simulink model "mainmodel"  (R2023b)
settings: Solver=FixedStepAuto  StartTime=0.0  StopTime=inf  RelTol=1e-3  EnableMultiTasking=on
libraries: vexarmcortexlib x26, simulink_extras x4, vexcommonlib x3
(part 2 of 2)

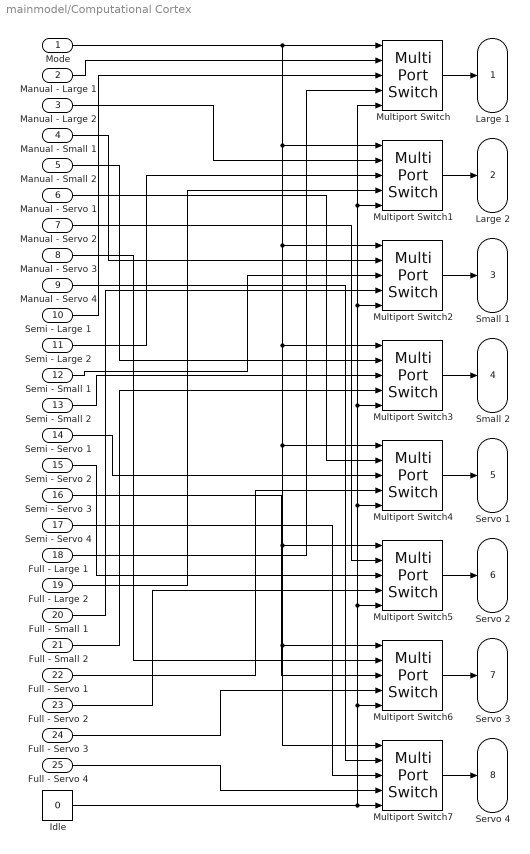
== system mainmodel/Computational Cortex ==
  Mode : Inport
  Manual - Large 1 : Inport  Port=2
  Manual - Large 2 : Inport  Port=3
  Manual - Small 1 : Inport  Port=4
  Manual - Small 2 : Inport  Port=5
  Manual - Servo 1 : Inport  Port=6
  Manual - Servo 2 : Inport  Port=7
  Manual - Servo 3 : Inport  Port=8
  Manual - Servo 4 : Inport  Port=9
  Semi - Large 1 : Inport  Port=10
  Semi - Large 2 : Inport  Port=11
  Semi - Small 1 : Inport  Port=12
  Semi - Small 2 : Inport  Port=13
  Semi - Servo 1 : Inport  Port=14
  Semi - Servo 2 : Inport  Port=15
  Semi - Servo 3 : Inport  Port=16
  Semi - Servo 4 : Inport  Port=17
  Full - Large 1 : Inport  Port=18
  Full - Large 2 : Inport  Port=19
  Full - Small 1 : Inport  Port=20
  Full - Small 2 : Inport  Port=21
  Full - Servo 1 : Inport  Port=22
  Full - Servo 2 : Inport  Port=23
  Full - Servo 3 : Inport  Port=24
  Full - Servo 4 : Inport  Port=25
  Idle : Constant  Value=0
  Multiport Switch{,1..7} (8 alike) : MultiPortSwitch  Inputs=4  SaturateOnIntegerOverflow=off  InputSameDT=off
  Large 1 : Outport
  Large 2 : Outport  Port=2
  Small 1 : Outport  Port=3
  Small 2 : Outport  Port=4
  Servo 1 : Outport  Port=5
  Servo 2 : Outport  Port=6
  Servo 3 : Outport  Port=7
  Servo 4 : Outport  Port=8
  wires:
  Multiport Switch/1 -> Large 1/1
  Multiport Switch1/1 -> Large 2/1
  Multiport Switch3/1 -> Small 2/1
  Multiport Switch2/1 -> Small 1/1
  Multiport Switch5/1 -> Servo 2/1
  Multiport Switch4/1 -> Servo 1/1
  Multiport Switch7/1 -> Servo 4/1
  Multiport Switch6/1 -> Servo 3/1
  Idle/1 -> Multiport Switch/5, Multiport Switch1/5, Multiport Switch2/5, Multiport Switch3/5, Multiport Switch4/5, Multiport Switch5/5, Multiport Switch6/5, Multiport Switch7/5
  Full - Servo 4/1 -> Multiport Switch7/4
  Full - Servo 3/1 -> Multiport Switch6/4
  Full - Servo 2/1 -> Multiport Switch5/4
  Full - Servo 1/1 -> Multiport Switch4/4
  Full - Small 2/1 -> Multiport Switch3/4
  Full - Small 1/1 -> Multiport Switch2/4
  Full - Large 2/1 -> Multiport Switch1/4
  Full - Large 1/1 -> Multiport Switch/4
  Semi - Servo 4/1 -> Multiport Switch7/3
  Semi - Servo 3/1 -> Multiport Switch6/3
  Semi - Servo 2/1 -> Multiport Switch5/3
  Semi - Servo 1/1 -> Multiport Switch4/3
  Semi - Small 2/1 -> Multiport Switch3/3
  Semi - Small 1/1 -> Multiport Switch2/3
  Semi - Large 2/1 -> Multiport Switch1/3
  Semi - Large 1/1 -> Multiport Switch/3
  Manual - Servo 4/1 -> Multiport Switch7/2
  Manual - Servo 3/1 -> Multiport Switch6/2
  Manual - Servo 2/1 -> Multiport Switch5/2
  Manual - Servo 1/1 -> Multiport Switch4/2
  Manual - Small 2/1 -> Multiport Switch3/2
  Manual - Small 1/1 -> Multiport Switch2/2
  Manual - Large 2/1 -> Multiport Switch1/2
  Manual - Large 1/1 -> Multiport Switch/2
  Mode/1 -> Multiport Switch3/1, Multiport Switch4/1, Multiport Switch7/1, Multiport Switch6/1, Multiport Switch5/1, Multiport Switch2/1, Multiport Switch1/1, Multiport Switch/1

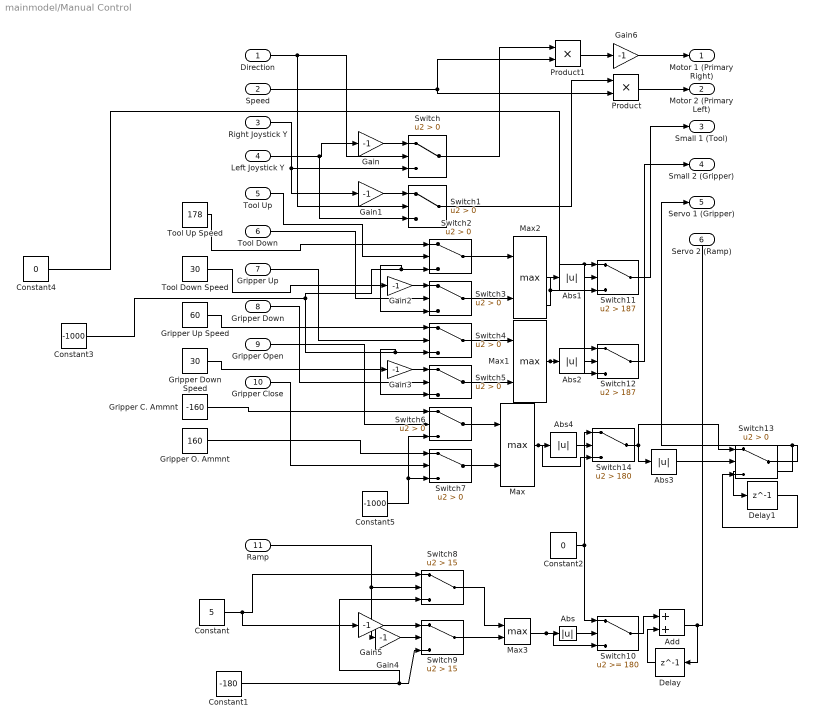
== system mainmodel/Manual Control ==
  Direction : Inport
  Speed : Inport  Port=2
  Right Joystick Y : Inport  Port=3
  Left Joystick Y : Inport  Port=4
  Tool Up : Inport  Port=5
  Tool Down : Inport  Port=6
  Gripper Up : Inport  Port=7
  Gripper Down : Inport  Port=8
  Gripper Open : Inport  Port=9
  Gripper Close : Inport  Port=10
  Ramp : Inport  Port=11
  Abs{,1..4} (5 alike) : Abs  SaturateOnIntegerOverflow=off
  Add : Sum
  Constant : Constant  Value=5
  Constant1 : Constant  Value=-180
  Constant2 : Constant  Value=0
  Constant3 : Constant  Value=-1000
  Constant4 : Constant  Value=0
  Constant5 : Constant  Value=-1000
  Delay : Delay  DelayLength=1
  Delay1 : Delay  DelayLength=1
  Gain{,1..6} (7 alike) : Gain  Gain=-1
  Gripper C. Ammnt : Constant  Value=-160
  Gripper Down Speed : Constant  Value=30
  Gripper O. Ammnt : Constant  Value=160
  Gripper Up Speed : Constant  Value=60
  Max{,1..3} (4 alike) : MinMax  Function=max  Inputs=2
  Product : Product  RndMeth=Zero
  Product1 : Product  RndMeth=Zero
  Switch{,1..7,13} (9 alike) : Switch  Criteria=u2 > Threshold  SaturateOnIntegerOverflow=off  InputSameDT=off
  Switch10 : Switch  Threshold=180  SaturateOnIntegerOverflow=off  InputSameDT=off
  Switch11 : Switch  Criteria=u2 > Threshold  Threshold=187  SaturateOnIntegerOverflow=off  InputSameDT=off
  Switch12 : Switch  Criteria=u2 > Threshold  Threshold=187  SaturateOnIntegerOverflow=off  InputSameDT=off
  Switch14 : Switch  Criteria=u2 > Threshold  Threshold=180  SaturateOnIntegerOverflow=off  InputSameDT=off
  Switch8 : Switch  Criteria=u2 > Threshold  Threshold=15  SaturateOnIntegerOverflow=off  InputSameDT=off
  Switch9 : Switch  Criteria=u2 > Threshold  Threshold=15  SaturateOnIntegerOverflow=off  InputSameDT=off
  Tool Down Speed : Constant  Value=30
  Tool Up Speed : Constant  Value=178
  Motor 1 (Primary Right) : Outport
  Motor 2 (Primary Left) : Outport  Port=2
  Small 1 (Tool) : Outport  Port=3
  Small 2 (Gripper) : Outport  Port=4
  Servo 1 (Gripper) : Outport  Port=5
  Servo 2 (Ramp) : Outport  Port=6
  wires:
  Gripper Close/1 -> Switch7/2
  Gripper Down Speed/1 -> Gain3/1
  Constant4/1 -> Switch12/1, Switch11/1
  Direction/1 -> Switch1/2, Switch/2
  Constant/1 -> Gain5/1, Switch8/1
  Tool Down/1 -> Switch3/2
  Delay1/1 -> Switch13/3
  Gripper C. Ammnt/1 -> Switch6/1
  Gain4/1 -> Switch9/2
  Max1/1 -> Switch12/3, Abs2/1
  Max3/1 -> Switch10/3, Abs/1
  Abs1/1 -> Switch11/2
  Tool Down Speed/1 -> Gain2/1
  Tool Up/1 -> Switch2/2
  Abs2/1 -> Switch12/2
  Max2/1 -> Abs1/1, Switch11/3
  Gain3/1 -> Switch5/1
  Switch9/1 -> Max3/2
  Constant3/1 -> Switch3/3, Switch2/3, Switch5/3, Switch4/3
  Switch6/1 -> Max/1
  Constant2/1 -> Switch10/1, Switch14/1
  Delay/1 -> Add/2
  Switch10/1 -> Add/1
  Gain5/1 -> Switch9/1
  Switch13/1 -> Servo 1 (Gripper)/1, Delay1/1
  Product/1 -> Motor 2 (Primary Left)/1
  Abs/1 -> Switch10/2
  Switch8/1 -> Max3/1
  Gain2/1 -> Switch3/1
  Ramp/1 -> Gain4/1, Switch8/2
  Add/1 -> Delay/1, Servo 2 (Ramp)/1
  Constant1/1 -> Switch8/3, Switch9/3
  Left Joystick Y/1 -> Switch1/3, Gain/1
  Switch/1 -> Product1/1
  Switch11/1 -> Small 1 (Tool)/1
  Gripper Down/1 -> Switch5/2
  Gripper Open/1 -> Switch6/2
  Tool Up Speed/1 -> Switch2/1
  Gripper Up/1 -> Switch4/2
  Switch12/1 -> Small 2 (Gripper)/1
  Switch7/1 -> Max/2
  Speed/1 -> Product/2, Product1/2
  Switch4/1 -> Max1/1
  Switch2/1 -> Max2/1
  Gripper O. Ammnt/1 -> Switch7/1
  Gripper Up Speed/1 -> Switch4/1
  Switch5/1 -> Max1/2
  Gain1/1 -> Switch1/1
  Switch3/1 -> Max2/2
  Right Joystick Y/1 -> Switch/3, Gain1/1
  Switch1/1 -> Product/1
  Gain/1 -> Switch/1
  Abs3/1 -> Switch13/2
  Constant5/1 -> Switch6/3, Switch7/3
  Max/1 -> Switch14/3, Abs4/1
  Abs4/1 -> Switch14/2
  Switch14/1 -> Abs3/1, Switch13/1
  Product1/1 -> Gain6/1
  Gain6/1 -> Motor 1 (Primary Right)/1

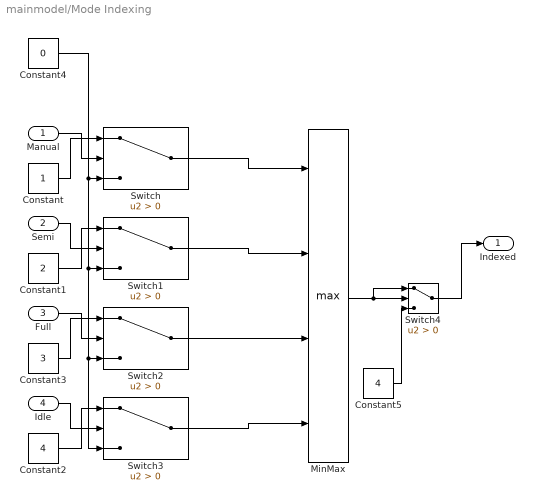
== system mainmodel/Mode Indexing ==
  Manual : Inport
  Semi : Inport  Port=2
  Full : Inport  Port=3
  Idle : Inport  Port=4
  Constant : Constant
  Constant1 : Constant  Value=2
  Constant2 : Constant  Value=4
  Constant3 : Constant  Value=3
  Constant4 : Constant  Value=0
  Constant5 : Constant  Value=4
  MinMax : MinMax  Function=max  Inputs=4
  Switch{,1..4} (5 alike) : Switch  Criteria=u2 > Threshold  SaturateOnIntegerOverflow=off  InputSameDT=off
  Indexed : Outport
  wires:
  Switch/1 -> MinMax/1
  Switch1/1 -> MinMax/2
  Switch2/1 -> MinMax/3
  Switch3/1 -> MinMax/4
  Manual/1 -> Switch/2
  Constant/1 -> Switch/1
  Constant1/1 -> Switch1/1
  Semi/1 -> Switch1/2
  Full/1 -> Switch2/2
  Constant3/1 -> Switch2/1
  Constant2/1 -> Switch3/1
  Idle/1 -> Switch3/2
  Constant4/1 -> Switch3/3, Switch2/3, Switch1/3, Switch/3
  MinMax/1 -> Switch4/1, Switch4/2
  Switch4/1 -> Indexed/1
  Constant5/1 -> Switch4/3

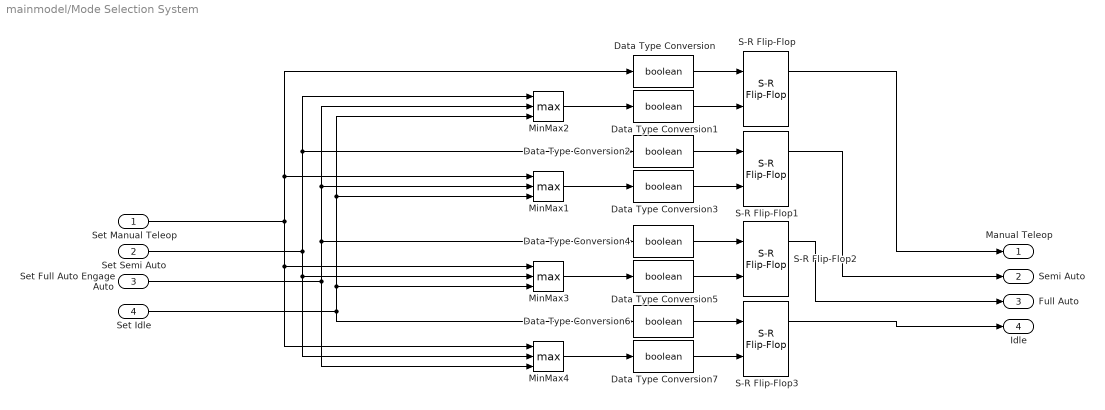
== system mainmodel/Mode Selection System ==
  Set Manual Teleop : Inport
  Set Semi Auto : Inport  Port=2
  Set Full Auto Engage Auto : Inport  Port=3
  Set Idle : Inport  Port=4
  Data Type Conversion{,1..7} (8 alike) : DataTypeConversion  OutDataTypeStr=boolean  ConvertRealWorld=Stored Integer (SI)  SaturateOnIntegerOverflow=off  RndMeth=Floor
  MinMax{1..4} (4 alike) : MinMax  Function=max  Inputs=3
  S-R Flip-Flop{,1..3} (4 alike) : simulink_extras/Flip Flops/S-R Flip-Flop  initial_condition=0
  Manual Teleop : Outport
  Semi Auto : Outport  Port=2
  Full Auto : Outport  Port=3
  Idle : Outport  Port=4
  wires:
  Set Semi Auto/1 -> MinMax3/2, MinMax4/2, MinMax2/1, Data Type Conversion2/1
  Set Full Auto Engage Auto/1 -> MinMax4/3, MinMax1/2, MinMax2/2, Data Type Conversion4/1
  Set Idle/1 -> Data Type Conversion6/1, MinMax3/3, MinMax1/3, MinMax2/3
  S-R Flip-Flop/1 -> Manual Teleop/1
  Data Type Conversion/1 -> S-R Flip-Flop/1
  Data Type Conversion1/1 -> S-R Flip-Flop/2
  MinMax2/1 -> Data Type Conversion1/1
  Set Manual Teleop/1 -> Data Type Conversion/1, MinMax1/1, MinMax3/1, MinMax4/1
  Data Type Conversion2/1 -> S-R Flip-Flop1/1
  MinMax1/1 -> Data Type Conversion3/1
  S-R Flip-Flop1/1 -> Semi Auto/1
  Data Type Conversion3/1 -> S-R Flip-Flop1/2
  Data Type Conversion4/1 -> S-R Flip-Flop2/1
  MinMax3/1 -> Data Type Conversion5/1
  S-R Flip-Flop2/1 -> Full Auto/1
  Data Type Conversion5/1 -> S-R Flip-Flop2/2
  Data Type Conversion6/1 -> S-R Flip-Flop3/1
  MinMax4/1 -> Data Type Conversion7/1
  S-R Flip-Flop3/1 -> Idle/1
  Data Type Conversion7/1 -> S-R Flip-Flop3/2

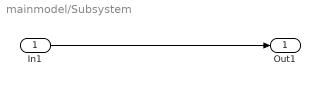
== system mainmodel/Subsystem ==
  In1 : Inport
  Out1 : Outport
  wires:
  In1/1 -> Out1/1

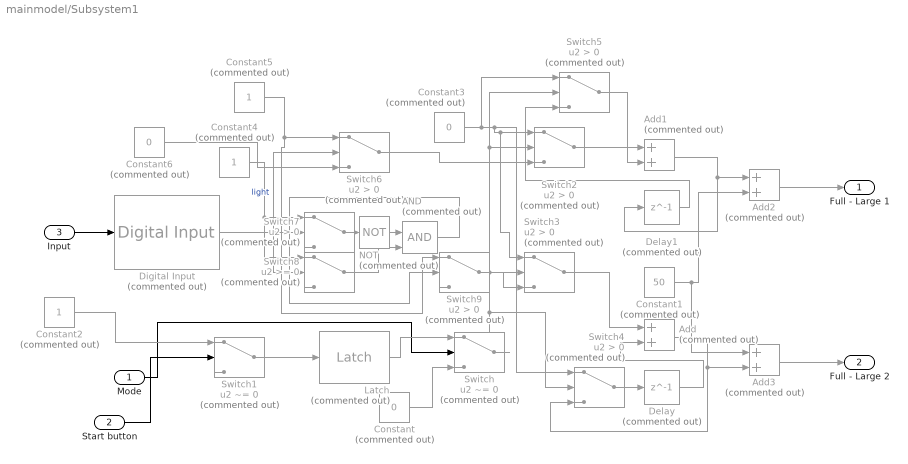
== system mainmodel/Subsystem1 ==
  " Mode" : Inport
  Start button : Inport  Port=2
  Input : Inport  Port=3
  AND : Logic  Commented=on  IconShape=distinctive  AllPortsSameDT=off  OutDataTypeStr=boolean
  Add{,1..3} (4 alike) : Sum  Commented=on
  Constant : Constant  Commented=on  Value=0
  Constant1 : Constant  Commented=on  Value=50
  Constant2 : Constant  Commented=on
  Constant3 : Constant  Commented=on  Value=0
  Constant4 : Constant  Commented=on
  Constant5 : Constant  Commented=on
  Constant6 : Constant  Commented=on  Value=0
  Delay : Delay  Commented=on  DelayLength=1
  Delay1 : Delay  Commented=on  DelayLength=1
  Digital Input : vexarmcortexlib/Sensors/Digital Input  Commented=on  inChan=1  SimulationIn=on  SampleTime=0.2
  Latch : vexcommonlib/Latch  Commented=on  output0=off  BlockPlatform=vexarmcortex
      settings: LibrarySourceBlock=vexarmcortexlib/Utilities/Latch
  NOT : Logic  Commented=on  Operator=NOT  IconShape=distinctive  AllPortsSameDT=off  OutDataTypeStr=boolean
  Switch : Switch  Commented=on  Criteria=u2 ~= 0  SaturateOnIntegerOverflow=off  InputSameDT=off
  Switch1 : Switch  Commented=on  Criteria=u2 ~= 0  SaturateOnIntegerOverflow=off  InputSameDT=off
  Switch{2..7,9} (7 alike) : Switch  Commented=on  Criteria=u2 > Threshold  SaturateOnIntegerOverflow=off  InputSameDT=off
  Switch8 : Switch  Commented=on  SaturateOnIntegerOverflow=off  InputSameDT=off
  Full - Large 1 : Outport
  Full - Large 2 : Outport  Port=2
  wires:
  Constant1/1 -> Add2/2, Add3/1
  Digital Input/1 -> Switch8/2, Switch6/2, Switch7/2  "light"
  Delay1/1 -> Switch5/3
  Delay/1 -> Add/2
  Add1/1 -> Add2/1, Delay1/1
  Add/1 -> Switch4/3, Add3/2
  Add2/1 -> Full - Large 1/1
  Add3/1 -> Full - Large 2/1
  Constant/1 -> Switch/3
  " Mode"/1 -> Switch/2
  Constant2/1 -> Switch1/1
  Latch/1 -> Switch/1
  Start button/1 -> Switch1/2
  Switch1/1 -> Latch/1
  Switch2/1 -> Add1/1
  Switch9/1 -> Switch3/3
  Switch/1 -> Switch5/2, Switch2/2, Switch3/2, Switch4/2
  Constant3/1 -> Switch5/1, Switch4/1, Switch2/1, Switch3/1
  Switch3/1 -> Add/1
  Switch4/1 -> Delay/1
  Switch5/1 -> Add1/2
  Input/1 -> Digital Input/1
  Switch7/1 -> NOT/1
  NOT/1 -> AND/1
  Switch8/1 -> AND/2
  AND/1 -> Switch9/2
  Constant5/1 -> Switch9/1, Switch6/1
  Switch6/1 -> Switch2/3
  Constant6/1 -> Switch6/3
  Constant4/1 -> Switch8/1, Switch7/1

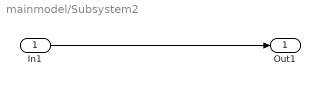
== system mainmodel/Subsystem2 ==
  In1 : Inport
  Out1 : Outport
  wires:
  In1/1 -> Out1/1
